simulink model "bh_mech_hardstop"  (R2017b)
settings: Solver=ode45  StartTime=0.0  StopTime=1  FixedStep=1e-4  MaxStep=1e-4  RelTol=1e-5
undefined symbols (not defined in the file): Mech, sigbuilder_block
settings Model: Creator=bhorton  LastModifiedBy=bhorton

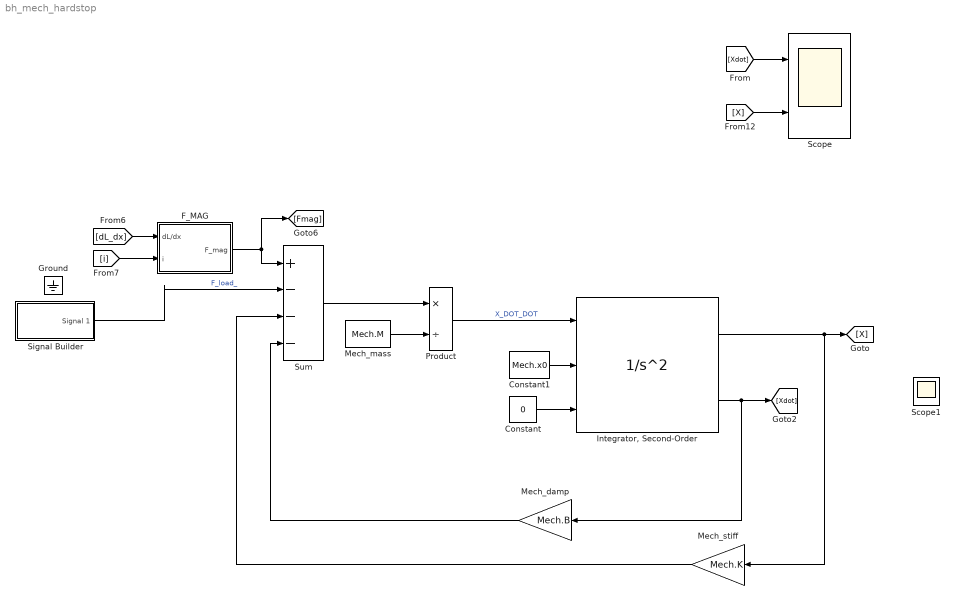
== system bh_mech_hardstop ==
  Constant : Constant  Value=0
  Constant1 : Constant  Value=Mech.x0
  F_MAG : Subsystem
  Ground : Ground
  "Integrator, Second-Order" : SecondOrderIntegrator  ICSourceX=external  LimitX=on  UpperLimitX=3e-3  LowerLimitX=-3e-3  ICSourceDXDT=external  ReinitDXDTwhenXreachesSaturation=on
  Mech_damp : Gain  Gain=Mech.B
  Mech_mass : Constant  Value=Mech.M
  Mech_stiff : Gain  Gain=Mech.K
  Product : Product  Inputs=*/
  Scope : Scope  NumInputPorts=2
  Scope1 : Scope
  Signal Builder : Subsystem  Tag=STV Subsys  LoadFcn=sigbuilder_block('load');  StartFcn=sigbuilder_block('start');  StopFcn=sigbuilder_block('stop');  ClipboardFcn=sigbuilder_block('clipboard');  mask(Sigbuilder block){tuvar=[0:10]}
      mask help: Simulink:masks:SigbuilderBlock_MD
      mask init:
      | if ~strcmp(get_param(bdroot(gcbh),'SimulationStatus'),'stopped') tuvar = sigbuilder_block('maskInit'); end
      settings: CopyFcn=sigbuilder_block('copy');  DeleteFcn=sigbuilder_block('delete');  ModelCloseFcn=sigbuilder_block('modelClose');  PreSaveFcn=sigbuilder_block('preSave');  PauseFcn=sigbuilder_block('pause');  ContinueFcn=sigbuilder_block('continue');  NameChangeFcn=sigbuilder_block('namechange');  OpenFcn=sigbuilder_block('open',[6 30 1428 681.75 ]);  CloseFcn=sigbuilder_block('close');
      mask Display: plot(0, 0, 100, 100,[2, 2, 32, 32, 2], [68, 8, 8, 68, 68],[32, 2], [38, 38], [32, 19, 2],[53, 60, 44], [32, 17, 17, 2],[16, 16, 31, 31]);txt = getActiveGroup(gcbh);text(2, 100, txt,'verticalAlignment', 'top');
  Sum : Sum  Inputs=+|-|-|-
  wires:
  Constant1/1 -> "Integrator, Second-Order"/2
  Constant/1 -> "Integrator, Second-Order"/3
  Sum/1 -> Product/1
  Mech_mass/1 -> Product/2
  Product/1 -> "Integrator, Second-Order"/1  "X_DOT_DOT"
  Mech_damp/1 -> Sum/4
  Mech_stiff/1 -> Sum/3
  Signal Builder/1(Signal 1) -> Sum/2  "F_load_"
  F_MAG/1(F_mag) -> [Fmag], Sum/1
  [dL_dx] -> F_MAG/1(dL/dx)
  [i] -> F_MAG/2(i)
  [X] -> Scope/2
  [Xdot] -> Scope/1
  "Integrator, Second-Order"/1 -> Mech_stiff/1, [X]
  "Integrator, Second-Order"/2 -> Mech_damp/1, [Xdot]

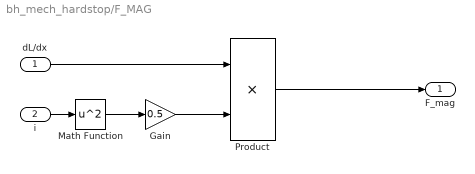
== system bh_mech_hardstop/F_MAG ==
  dL/dx : Inport
  i : Inport  Port=2
  Gain : Gain  Gain=0.5
  Math Function : Math  Operator=square  SaturateOnIntegerOverflow=on
  Product : Product
  F_mag : Outport
  wires:
  Product/1 -> F_mag/1
  i/1 -> Math Function/1
  Math Function/1 -> Gain/1
  dL/dx/1 -> Product/1
  Gain/1 -> Product/2

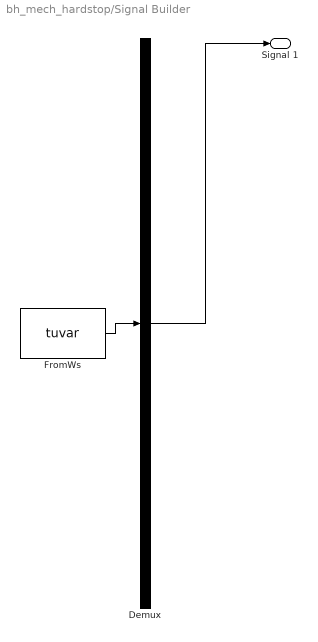
== system bh_mech_hardstop/Signal Builder ==
  Demux : Demux  Tag=STV Demux  Outputs=1
  FromWs : FromWorkspace  Tag=STV FromWs  VariableName=tuvar  SampleTime=0
      SigBuilderData=|
      | common.afterFinalStr = 'Extrapolate'
      | common.sampleTime = 0
      | dataSet.timeRange = [0 10]
      | dataSet.name = 'Group 1'
      | sbobj.Groups.Name = 'Group 1'
      | sbobj.Groups.Signals.Name = 'Signal 1'
      | sbobj.Groups.Signals.XData = [0 0.4 0.4 0.7 0.7 10]
      | sbobj.Groups.Signals.YData = [0 0 10 10 0 0]
  Signal 1 : Outport  Tag=STV Outport
  wires:
  Demux/1 -> Signal 1/1
  FromWs/1 -> Demux/1
